simulink model "PWM_module"  (R2015b)
settings: Solver=VariableStepAuto  StartTime=0.0  StopTime=inf  RelTol=1e-3
libraries: powerlib x12, powerlib_meascontrol x1
settings Model: Creator=shangwei  LastModifiedBy=root

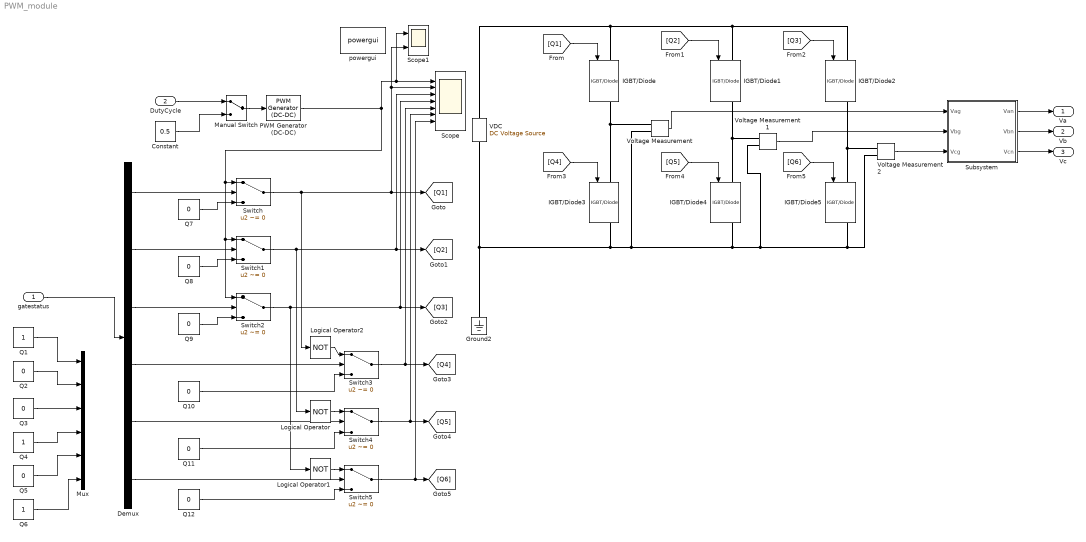
== system PWM_module ==
  gatestatus : Inport
  DutyCycle : Inport  Port=2
  Constant : Constant  Value=0.5
  Demux : Demux  Outputs=6
  Ground2 : powerlib/Elements/Ground  LConnTagsString=a
  IGBT/Diode{,1..5} (6 alike) : powerlib/Power Electronics/IGBT//Diode  Ron=1e-3  Rs=1e5  Cs=inf  Measurements=on
  Logical Operator : Logic  Operator=NOT  AllPortsSameDT=off  OutDataTypeStr=boolean
  Logical Operator1 : Logic  Operator=NOT  AllPortsSameDT=off  OutDataTypeStr=boolean
  Logical Operator2 : Logic  Operator=NOT  AllPortsSameDT=off  OutDataTypeStr=boolean
  Manual Switch : ManualSwitch
  Mux : Mux  Inputs=6
  PWM Generator (DC-DC) : powerlib_meascontrol/Pulse & Signal Generators/PWM Generator (DC-DC)  Fsw=5000  Ts=0
  Q1 : Constant
  Q{2..3,5,7..12} (9 alike) : Constant  Value=0
  Q4 : Constant
  Q6 : Constant
  Scope : Scope  NumInputPorts=7
  Scope1 : Scope  NumInputPorts=2
  Subsystem : Subsystem
  Switch{,1..5} (6 alike) : Switch  Criteria=u2 ~= 0
  VDC : powerlib/Electrical Sources/DC Voltage Source  Amplitude=24  Measurements=Voltage
  Voltage Measurement : powerlib/Measurements/Voltage Measurement  PhasorSimulation=off  OutputType=Complex  PSBequivalent=0
  Voltage Measurement1 : powerlib/Measurements/Voltage Measurement  PhasorSimulation=off  OutputType=Complex  PSBequivalent=0
  Voltage Measurement2 : powerlib/Measurements/Voltage Measurement  PhasorSimulation=off  OutputType=Complex  PSBequivalent=0
  powergui : powerlib/powergui  Priority=1  SimulationMode=Discrete  SolverType=Tustin/Backward Euler (TBE)  SampleTime=50e-2  frequency=60  SPID=off  DisableSnubberDevices=off  DisableRonSwitches=off  DisableVfSwitches=off  SwTol=0  DisplayEquations=off  Interpol=off  ExternalGateDelay=off  methode=off  Ts=10  FunctionMessages=off  echomessages=off  HookPort=off  EnableUseOfTLC=off  x0status=blocks  frequencyindice=0  Pbase=100e6  ErrMax=1e-4  Iterations=50  UnitsV=kV  UnitsW=MW  buscounter=0  RestoreLinks=warning  ResistiveCurrentMeasurement=off  Frange=[0:2:500]  Ylog=off  Xlog=on  ShowGrid=off  save=off  variable=ZData  structure=0  ZoomFFT=off  StartTime=0.0  cycles=1  DisplayStyle=1  fundamental=60  FreqAxis=off  MaxFrequency=1000  frequencyindicesteady=1  RmsSteady=1  display=off
  Va : Outport
  Vb : Outport  Port=2
  Vc : Outport  Port=3
  wires:
  [Q2] -> IGBT/Diode1/1
  [Q3] -> IGBT/Diode2/1
  [Q4] -> IGBT/Diode3/1
  [Q5] -> IGBT/Diode4/1
  [Q6] -> IGBT/Diode5/1
  Voltage Measurement/1 -> Subsystem/1(Vag)
  Voltage Measurement1/1 -> Subsystem/2(Vbg)
  Voltage Measurement2/1 -> Subsystem/3(Vcg)
  Subsystem/1(Van) -> Va/1
  Subsystem/2(Vbn) -> Vb/1
  Subsystem/3(Vcn) -> Vc/1
  PWM Generator (DC-DC)/1 -> Switch2/1, Switch1/1, Switch/1, Scope1/1, Scope/1
  Demux/1 -> Switch/2
  Switch/1 -> Logical Operator2/1, Scope1/2, Scope/2, [Q1]
  Demux/2 -> Switch1/2
  Switch1/1 -> Logical Operator/1, Scope/3, [Q2]
  Demux/3 -> Switch2/2
  Switch2/1 -> Logical Operator1/1, Scope/4, [Q3]
  Demux/4 -> Switch3/2
  Demux/5 -> Switch4/2
  Demux/6 -> Switch5/2
  DutyCycle/1 -> Manual Switch/1
  Manual Switch/1 -> PWM Generator (DC-DC)/1
  Constant/1 -> Manual Switch/2
  gatestatus/1 -> Demux/1
  Q1/1 -> Mux/1
  Q2/1 -> Mux/2
  Q3/1 -> Mux/3
  Q4/1 -> Mux/4
  Q5/1 -> Mux/5
  Q6/1 -> Mux/6
  Q7/1 -> Switch/3
  Q8/1 -> Switch1/3
  Q9/1 -> Switch2/3
  Q10/1 -> Switch3/3
  Q11/1 -> Switch4/3
  Q12/1 -> Switch5/3
  Switch3/1 -> Scope/5, [Q4]
  Switch4/1 -> Scope/6, [Q5]
  Switch5/1 -> Scope/7, [Q6]
  Logical Operator2/1 -> Switch3/1
  Logical Operator/1 -> Switch4/1
  Logical Operator1/1 -> Switch5/1
  [Q1] -> IGBT/Diode/1
  connections:
  IGBT/Diode/RConn1 -- Voltage Measurement/LConn1 -- IGBT/Diode3/LConn1
  IGBT/Diode1/RConn1 -- Voltage Measurement1/LConn1 -- IGBT/Diode4/LConn1
  IGBT/Diode2/RConn1 -- Voltage Measurement2/LConn1 -- IGBT/Diode5/LConn1
  VDC/RConn1 -- IGBT/Diode2/LConn1 -- IGBT/Diode1/LConn1 -- IGBT/Diode/LConn1
  VDC/LConn1 -- Ground2/LConn1 -- Voltage Measurement/LConn2 -- IGBT/Diode4/RConn1 -- Voltage Measurement2/LConn2 -- IGBT/Diode5/RConn1 -- Voltage Measurement1/LConn2 -- IGBT/Diode3/RConn1

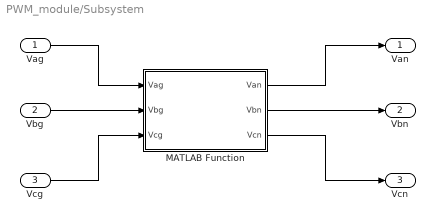
== system PWM_module/Subsystem ==
  Vag : Inport
  Vbg : Inport  Port=2
  Vcg : Inport  Port=3
  MATLAB Function : MATLAB Function  TreatAsAtomicUnit=on
  Van : Outport
  Vbn : Outport  Port=2
  Vcn : Outport  Port=3
  wires:
  Vag/1 -> MATLAB Function/1(Vag)
  Vbg/1 -> MATLAB Function/2(Vbg)
  Vcg/1 -> MATLAB Function/3(Vcg)
  MATLAB Function/1(Van) -> Van/1
  MATLAB Function/2(Vbn) -> Vbn/1
  MATLAB Function/3(Vcn) -> Vcn/1

== matlab function PWM_module/Subsystem/MATLAB Function ==
  data: Vag input; Van output; Vbg input; Vcg input; Vbn output; Vcn output
function [Van, Vbn, Vcn] = poletophase(Vag, Vbg, Vcg)
%%#codegen
Trans = [ 2/3 -1/3 -1/3 ; -1/3 2/3 -1/3 ; -1/3 -1/3 2/3];

u = [Vag; Vbg; Vcg];
y = Trans * u ;
Van = y(1);
Vbn = y(2);
Vcn = y(3);

%% according to the technical report written by Ti
% http://www.ti.com/lit/an/spra498/spra498.pdf
% Trans = [ 1/3 1/3 1/3 ; 1/3 1/3 1/3 ; 1/3 1/3 1/3];
% 
% u = [Vag; Vbg; Vcg];
% y = Trans * u ;
% Van = y(1);
% Vbn = y(2);
% Vcn = y(3);

%%
